simulink model "FinalTest_21_3_Duy"  (R2019b)
settings: Solver=VariableStepAuto  StartTime=0.0  StopTime=10.0  RelTol=1e-3
undefined symbols (not defined in the file): G, Rollingresistancecoefficient
libraries: simulink_extras x4, vehdynlibsteering x1, autolibshared x1
settings Model: Creator=Lenovo  LastModifiedBy=Lenovo
settings DebuggingCC: UnconnectedInputMsg=none  UnconnectedOutputMsg=none  UnconnectedLineMsg=none  SFMachineParentedDataDiag=error
settings ModelReferenceCC: EnableRefExpFcnMdlSchedulingChecks=off
settings RTWCC: Description=Generic Real-Time Target

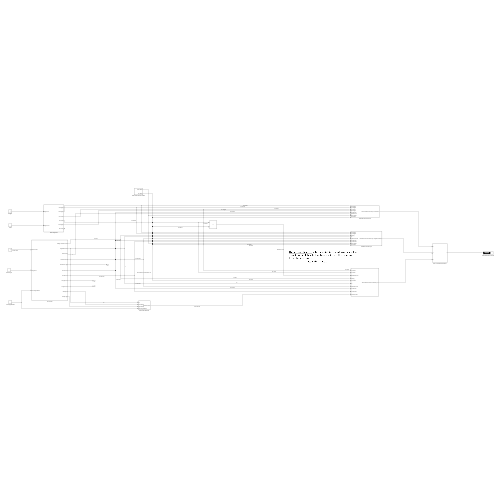
[thumbnail: Simulink's stored preview of the top-level diagram]
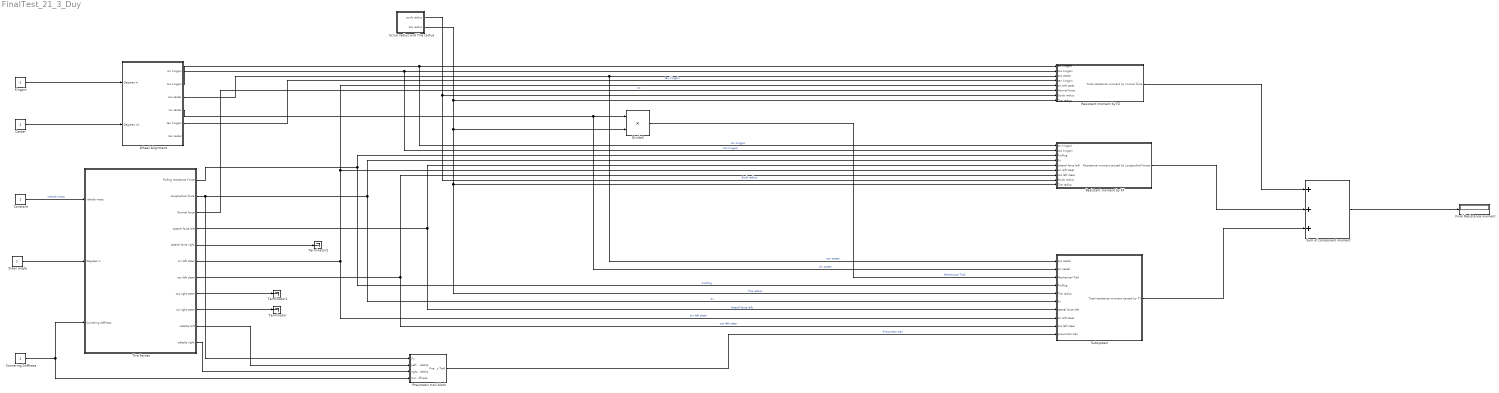
== system FinalTest_21_3_Duy ==
  Caster : Constant
  Constant : Constant
  Cornering Stiffness : Constant
  Divide2 : Product  Inputs=**
  Final Resistance moment : Display
  Kingpin : Constant
  Pneumatic trail block : Subsystem
  Resistant moment by FX : Subsystem
  Resistant moment by FZ : Subsystem
  Scrub radius and Tire radius : Subsystem
  Steer angle : Constant
  Subsystem : Subsystem
  Sum of component moment : Sum  Inputs=+++
  Terminator : Terminator
  Terminator1 : Terminator
  Terminator2 : Terminator
  Tire Forces : Subsystem
  Wheel Alignment : Subsystem
  wires:
  Constant/1 -> Tire Forces/1(vehicle mass)  "vehicle mass"
  Steer angle/1 -> Tire Forces/2(Degrees in)
  Tire Forces/3(Normal force) -> Resistant moment by FZ/6(Normal force)  "Fz"
  Tire Forces/5(Lateral force right) -> Terminator2/1
  Tire Forces/8(cos right steer) -> Terminator1/1
  Tire Forces/9(sin right steer) -> Terminator/1
  Kingpin/1 -> Wheel Alignment/1(Degrees in)
  Caster/1 -> Wheel Alignment/2(Degrees in1)
  Wheel Alignment/4(sin caster) -> Subsystem/2(sin caster), Divide2/1  "sin caster"
  Wheel Alignment/1(sin kingpin) -> Resistant moment by FX/1(sin kingpin), Resistant moment by FZ/1(sin kingpin)  "sin kingpin"
  Wheel Alignment/2(cos kingpin) -> Resistant moment by FX/2(cos kingpin), Resistant moment by FZ/2(cos kingpin)  "cos kingpin"
  Wheel Alignment/3(cos caster) -> Subsystem/1(cos caster), Resistant moment by FZ/3(cos caster)  "cos caster"
  Wheel Alignment/5(tan kingpin) -> Resistant moment by FZ/4(tan kingpin)  "tan kingpin"
  Tire Forces/6(sin left steer) -> Subsystem/8(sin left steer), Resistant moment by FZ/5(sin left steer), Resistant moment by FX/6(sin left steer)  "sin left steer"
  Tire Forces/1(Rolling resistance Force) -> Subsystem/4(Frolling), Resistant moment by FX/3(Frolling)  "Frolling"
  Tire Forces/2(Longitudinal force) -> Pneumatic trail block/1(Fx), Subsystem/6(Fx), Resistant moment by FX/4(Fx)  "Fx"
  Tire Forces/4(Lateral force left) -> Subsystem/7(lateral force left), Resistant moment by FX/5(Lateral force left)  "lateral force left"
  Tire Forces/7(cos left steer) -> Subsystem/9(cos left steer), Resistant moment by FX/7(cos left steer)  "cos left steer"
  Cornering Stiffness/1 -> Pneumatic trail block/4(Cornering Stiffness), Tire Forces/3(Cornering stiffness)
  Tire Forces/10(sidelsip left) -> Pneumatic trail block/2(Left sideslip)
  Tire Forces/11(sideslip right) -> Pneumatic trail block/3(right sideslip)
  Scrub radius and Tire radius/2(tire radius) -> Subsystem/5(Tire radius), Resistant moment by FX/9(Tire radius), Divide2/2, Resistant moment by FZ/8(Tire radius)  "Tire radius"
  Scrub radius and Tire radius/1(scrub radius) -> Resistant moment by FX/8(Scrub radius), Resistant moment by FZ/7(Scrub radius)  "Scub radius"
  Divide2/1 -> Subsystem/3(Mechanical Trail)  "Mechanical Trail"
  Pneumatic trail block/1(Pneumatic Trail) -> Subsystem/10(pneumatic trail)  "Pneumatic trail"
  Resistant moment by FZ/1(Toral resistance moment by normal force) -> Sum of component moment/1
  Subsystem/1(Total resistance moment caused by FY) -> Sum of component moment/3
  Resistant moment by FX/1(Resistance moment caused by Longitudinal forces) -> Sum of component moment/2
  Sum of component moment/1 -> Final Resistance moment/1

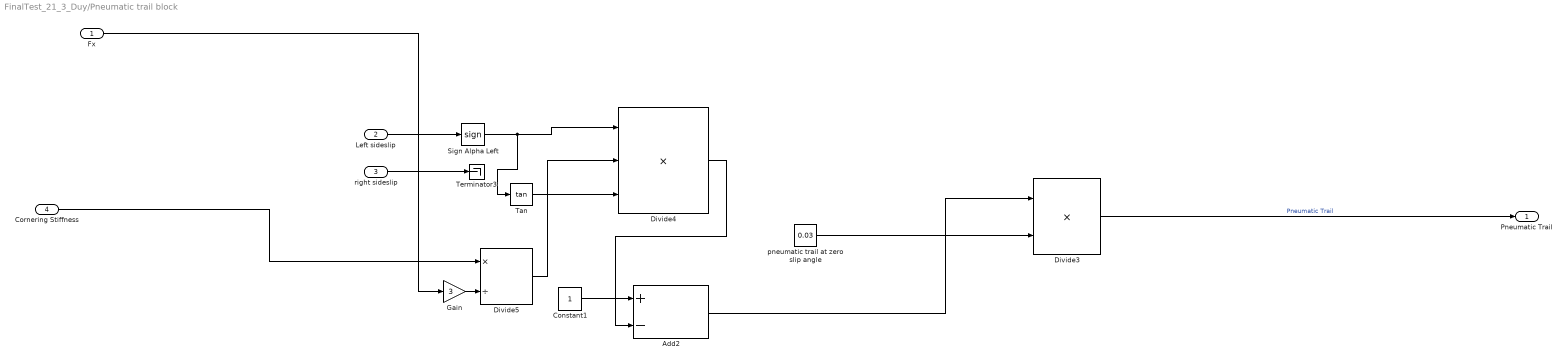
== system FinalTest_21_3_Duy/Pneumatic trail block ==
  Fx : Inport
  Left sideslip : Inport  Port=2
  right sideslip : Inport  Port=3
  Cornering Stiffness : Inport  Port=4
  Add2 : Sum  Inputs=+-
  Constant1 : Constant
  Divide3 : Product  Inputs=**
  Divide4 : Product  Inputs=***
  Divide5 : Product  Inputs=*/
  Gain : Gain  Gain=3
  Sign Alpha Left : Signum
  Tan : Trigonometry  Operator=tan
  Terminator3 : Terminator
  pneumatic trail at zero slip angle : Constant  Value=0.03
  Pneumatic Trail : Outport
  wires:
  Constant1/1 -> Add2/1
  Divide4/1 -> Add2/2
  Divide5/1 -> Divide4/2
  Tan/1 -> Divide4/3
  Sign Alpha Left/1 -> Tan/1, Divide4/1
  pneumatic trail at zero slip angle/1 -> Divide3/2
  Gain/1 -> Divide5/2
  Add2/1 -> Divide3/1
  Left sideslip/1 -> Sign Alpha Left/1
  Divide3/1 -> Pneumatic Trail/1  "Pneumatic Trail"
  right sideslip/1 -> Terminator3/1
  Fx/1 -> Gain/1
  Cornering Stiffness/1 -> Divide5/1

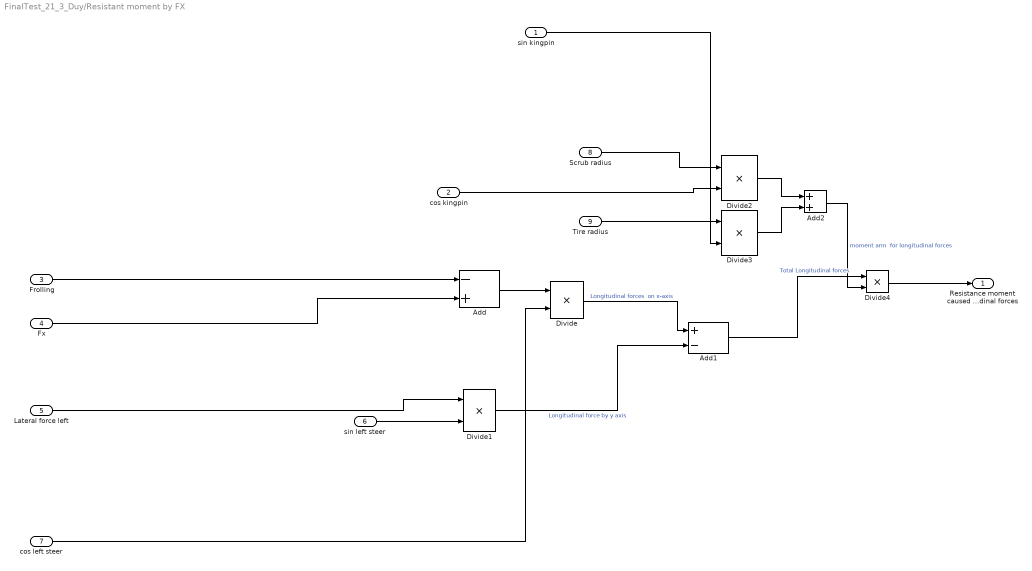
== system FinalTest_21_3_Duy/Resistant moment by FX ==
  sin kingpin : Inport
  cos kingpin : Inport  Port=2
  Frolling : Inport  Port=3
  Fx : Inport  Port=4
  Lateral force left : Inport  Port=5
  sin left steer : Inport  Port=6
  cos left steer : Inport  Port=7
  Scrub radius : Inport  Port=8
  Tire radius : Inport  Port=9
  Add : Sum  Inputs=-+
  Add1 : Sum  Inputs=+-
  Add2 : Sum
  Divide{,1..4} (5 alike) : Product  Inputs=**
  Resistance moment caused by Longitudinal forces : Outport
  wires:
  Scrub radius/1 -> Divide2/1
  Add1/1 -> Divide4/1  "Total Longitudinal forces"
  Divide/1 -> Add1/1  "Longitudinal forces  on x-axis"
  Divide1/1 -> Add1/2  "Longitudinal force by y axis"
  Lateral force left/1 -> Divide1/1
  Add/1 -> Divide/1
  Add2/1 -> Divide4/2  "moment arm  for longitudinal forces"
  Divide4/1 -> Resistance moment caused by Longitudinal forces/1
  Divide2/1 -> Add2/1
  Tire radius/1 -> Divide3/1
  Divide3/1 -> Add2/2
  cos kingpin/1 -> Divide2/2
  cos left steer/1 -> Divide/2
  sin left steer/1 -> Divide1/2
  Fx/1 -> Add/2
  Frolling/1 -> Add/1
  sin kingpin/1 -> Divide3/2

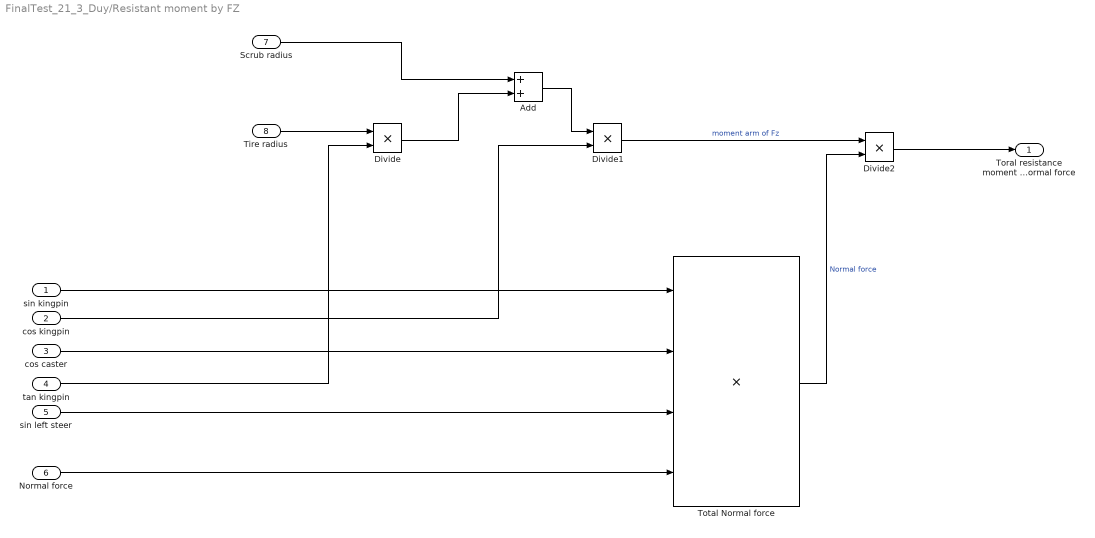
== system FinalTest_21_3_Duy/Resistant moment by FZ ==
  sin kingpin : Inport
  cos kingpin : Inport  Port=2
  cos caster : Inport  Port=3
  tan kingpin : Inport  Port=4
  sin left steer : Inport  Port=5
  Normal force : Inport  Port=6
  Scrub radius : Inport  Port=7
  Tire radius : Inport  Port=8
  Add : Sum
  Divide : Product  Inputs=**
  Divide1 : Product  Inputs=**
  Divide2 : Product  Inputs=**
  Total Normal force : Product  Inputs=****
  Toral resistance moment by normal force : Outport
  wires:
  Tire radius/1 -> Divide/1
  cos kingpin/1 -> Divide1/2
  sin kingpin/1 -> Total Normal force/1
  Scrub radius/1 -> Add/1
  Total Normal force/1 -> Divide2/2  "Normal force"
  Divide1/1 -> Divide2/1  "moment arm of Fz"
  Divide/1 -> Add/2
  Add/1 -> Divide1/1
  cos caster/1 -> Total Normal force/2
  sin left steer/1 -> Total Normal force/3
  tan kingpin/1 -> Divide/2
  Divide2/1 -> Toral resistance moment by normal force/1
  Normal force/1 -> Total Normal force/4

== system FinalTest_21_3_Duy/Scrub radius and Tire radius ==
  Scrub radius : Constant
  Tire radius : Constant
  scrub radius : Outport
  tire radius : Outport  Port=2
  wires:
  Tire radius/1 -> tire radius/1  "tire radius"
  Scrub radius/1 -> scrub radius/1  "scrub radius"

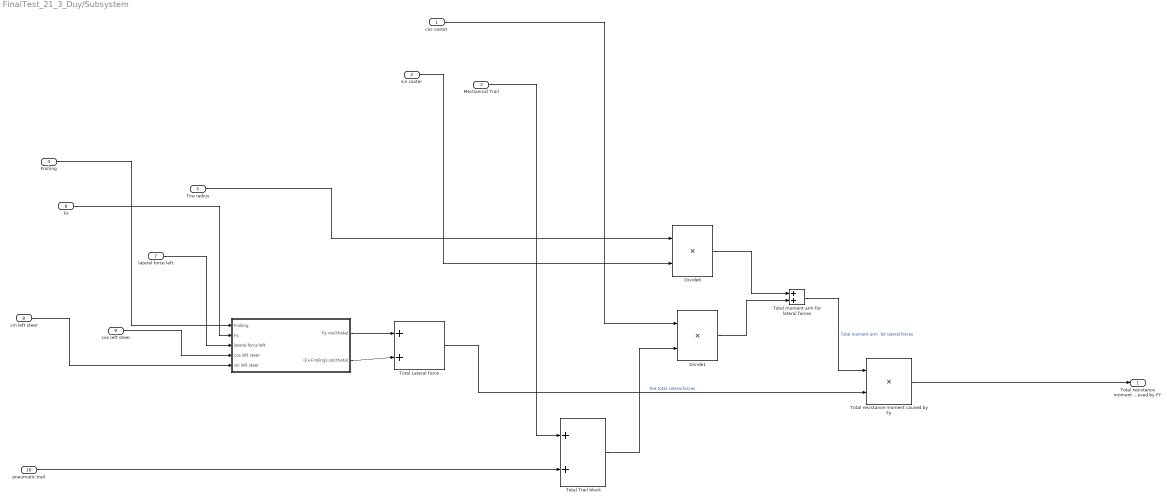
== system FinalTest_21_3_Duy/Subsystem ==
  cos caster : Inport
  sin caster : Inport  Port=2
  Mechanical Trail : Inport  Port=3
  Frolling : Inport  Port=4
  Tire radius : Inport  Port=5
  Fx : Inport  Port=6
  lateral force left : Inport  Port=7
  sin left steer : Inport  Port=8
  cos left steer : Inport  Port=9
  pneumatic trail : Inport  Port=10
  " " : Subsystem
  Divide1 : Product  Inputs=**
  Divide6 : Product  Inputs=**
  Total Lateral force : Sum
  Total Trail block : Sum
  Total moment arm for lateral forces : Sum
  Total resistance moment caused by Fy : Product  Inputs=**
  Total resistance moment caused by FY : Outport
  wires:
  cos caster/1 -> Divide1/1
  Divide6/1 -> Total moment arm for lateral forces/1
  Total moment arm for lateral forces/1 -> Total resistance moment caused by Fy/1  "Total moment arm  for lateral forces"
  Total Lateral force/1 -> Total resistance moment caused by Fy/2  "the total  lateral forces"
  Divide1/1 -> Total moment arm for lateral forces/2
  " "/1(Fy.cos(theta)) -> Total Lateral force/1
  Total Trail block/1 -> Divide1/2
  " "/2((Fx-Frolling).sin(theta)) -> Total Lateral force/2
  Total resistance moment caused by Fy/1 -> Total resistance moment caused by FY/1
  pneumatic trail/1 -> Total Trail block/2
  Tire radius/1 -> Divide6/1
  sin caster/1 -> Divide6/2
  cos left steer/1 -> " "/4(cos left steer)
  Frolling/1 -> " "/1(Frolling)
  lateral force left/1 -> " "/3(lateral force left)
  sin left steer/1 -> " "/5(sin left steer)
  Fx/1 -> " "/2(Fx)
  Mechanical Trail/1 -> Total Trail block/1

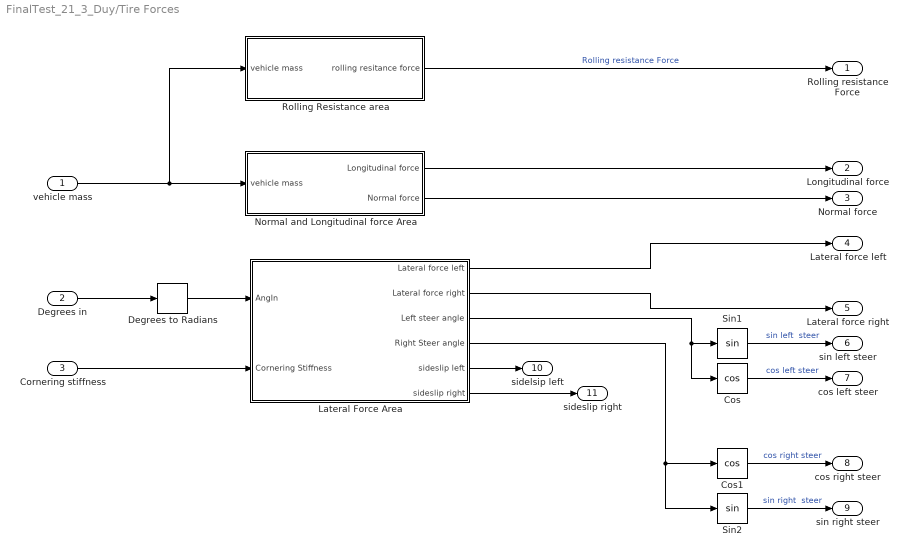
== system FinalTest_21_3_Duy/Tire Forces ==
  vehicle mass : Inport
  Degrees in : Inport  Port=2
  Cornering stiffness : Inport  Port=3
  Cos : Trigonometry  Operator=cos
  Cos1 : Trigonometry  Operator=cos
  Degrees to Radians : simulink_extras/Transformations/Degrees to Radians
  Lateral Force Area : Subsystem
  Normal and Longitudinal force Area : Subsystem
  Rolling Resistance area : Subsystem
  Sin1 : Trigonometry
  Sin2 : Trigonometry
  Rolling resistance Force : Outport
  Longitudinal force : Outport  Port=2
  Normal force : Outport  Port=3
  Lateral force left : Outport  Port=4
  Lateral force right : Outport  Port=5
  sin left steer : Outport  Port=6
  cos left steer : Outport  Port=7
  cos right steer : Outport  Port=8
  sin right steer : Outport  Port=9
  sidelsip left : Outport  Port=10
  sideslip right : Outport  Port=11
  wires:
  Degrees to Radians/1 -> Lateral Force Area/1(AngIn)
  Lateral Force Area/4(Right Steer angle) -> Sin2/1, Cos1/1
  vehicle mass/1 -> Rolling Resistance area/1(vehicle mass), Normal and Longitudinal force Area/1(vehicle mass)
  Sin2/1 -> sin right steer/1  "sin right  steer"
  Cos1/1 -> cos right steer/1  "cos right steer"
  Lateral Force Area/3(Left steer angle) -> Sin1/1, Cos/1
  Normal and Longitudinal force Area/1(Longitudinal force) -> Longitudinal force/1
  Normal and Longitudinal force Area/2(Normal force) -> Normal force/1
  Sin1/1 -> sin left steer/1  "sin left  steer"
  Rolling Resistance area/1(rolling resitance force) -> Rolling resistance Force/1  "Rolling resistance Force"
  Degrees in/1 -> Degrees to Radians/1
  Cos/1 -> cos left steer/1  "cos left steer"
  Lateral Force Area/2(Lateral force right) -> Lateral force right/1
  Lateral Force Area/1(Lateral force left) -> Lateral force left/1
  Lateral Force Area/5(sideslip left) -> sidelsip left/1
  Lateral Force Area/6("sideslip right ") -> sideslip right/1
  Cornering stiffness/1 -> Lateral Force Area/2(Cornering Stiffness)

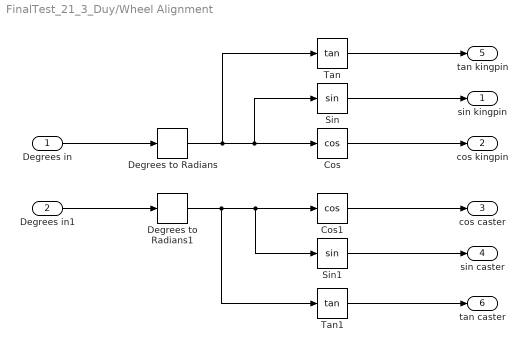
== system FinalTest_21_3_Duy/Wheel Alignment ==
  Degrees in : Inport
  Degrees in1 : Inport  Port=2
  Cos : Trigonometry  Operator=cos
  Cos1 : Trigonometry  Operator=cos
  Degrees to Radians : simulink_extras/Transformations/Degrees to Radians
  Degrees to Radians1 : simulink_extras/Transformations/Degrees to Radians
  Sin : Trigonometry
  Sin1 : Trigonometry
  Tan : Trigonometry  Operator=tan
  Tan1 : Trigonometry  Operator=tan
  sin kingpin : Outport
  cos kingpin : Outport  Port=2
  cos caster : Outport  Port=3
  sin caster : Outport  Port=4
  tan kingpin : Outport  Port=5
  tan caster : Outport  Port=6
  wires:
  Sin1/1 -> sin caster/1
  Degrees to Radians1/1 -> Tan1/1, Sin1/1, Cos1/1
  Sin/1 -> sin kingpin/1
  Degrees in1/1 -> Degrees to Radians1/1
  Cos1/1 -> cos caster/1
  Cos/1 -> cos kingpin/1
  Degrees to Radians/1 -> Tan/1, Sin/1, Cos/1
  Degrees in/1 -> Degrees to Radians/1
  Tan/1 -> tan kingpin/1
  Tan1/1 -> tan caster/1

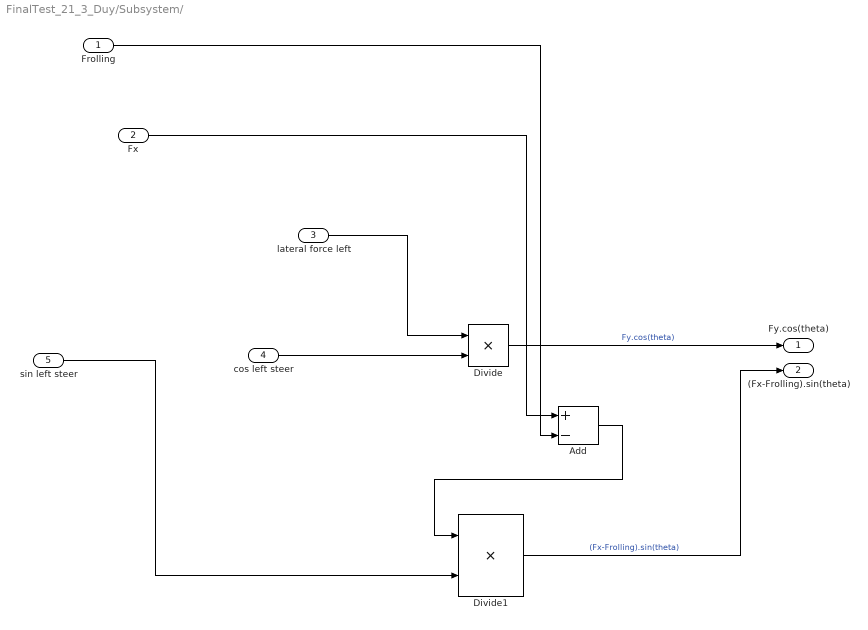
== system FinalTest_21_3_Duy/Subsystem/  ==
  Frolling : Inport
  Fx : Inport  Port=2
  lateral force left : Inport  Port=3
  cos left steer : Inport  Port=4
  sin left steer : Inport  Port=5
  Add : Sum  Inputs=+-
  Divide : Product  Inputs=**
  Divide1 : Product  Inputs=**
  Fy.cos(theta) : Outport
  (Fx-Frolling).sin(theta) : Outport  Port=2
  wires:
  Divide1/1 -> (Fx-Frolling).sin(theta)/1  "(Fx-Frolling).sin(theta)"
  Add/1 -> Divide1/1
  Frolling/1 -> Add/2
  lateral force left/1 -> Divide/1
  cos left steer/1 -> Divide/2
  sin left steer/1 -> Divide1/2
  Fx/1 -> Add/1
  Divide/1 -> Fy.cos(theta)/1  "Fy.cos(theta)"

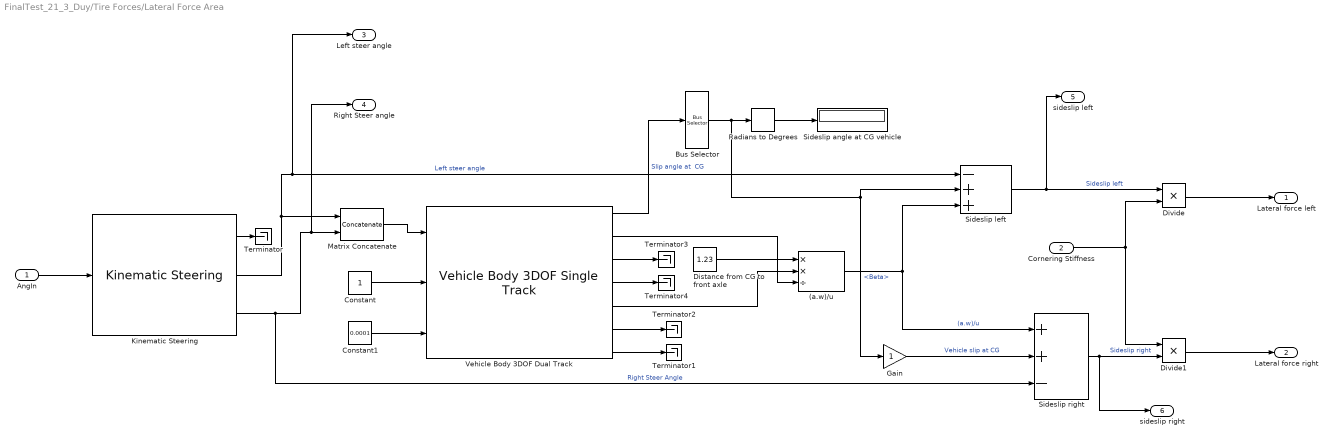
== system FinalTest_21_3_Duy/Tire Forces/Lateral Force Area ==
  AngIn : Inport
  Cornering Stiffness : Inport  Port=2
  (a.w)/u : Product  Inputs=**/
  Bus Selector : BusSelector  OutputSignals=BdyFrm.Cg.Ang.Beta
  Constant : Constant
  Constant1 : Constant  Value=0.0001
  Distance from CG to front axle : Constant  Value=1.23
  Divide : Product  Inputs=**
  Divide1 : Product  Inputs=**
  Gain : Gain
  Kinematic Steering : vehdynlibsteering/Kinematic Steering  StrgType=Rack and pinion  StrgRatioType=Constant  Loc=Front  NrmlFctr=0.01  TrckWdth=1.475  WhlBase=1.524  Db=0  StrgRng=6*pi  StrgAngBpts="[-6.2832   -5.0265   -3.7699   -2.5133   -1.2566         0    1.2566    2.5133    3.7699    5.0265    6.2832]"  StrgRatioTbl=|  StrgRatio=100  PctAckIn=off  PctAck=100  PctAckTbl=ones(1,11)*100  StrgArmLngth=0.3  RckCsLngth=0.65  TieRodLngth=0.13  D=0.12  PnnRadius=0.007  PnnRadiusTbl="[0.0055    0.0055    0.0056    0.0057    0.0058    0.0057    0.0057    0.0057    0.0056    0.0055    0.0055]"  RodLngth=0.1  ParaArmLngth=0.9  aMode=2
      | [13.5000   13.3750   13.2500   13.1250   13.0000   13.0000   13.0000   13.1250   13.2500   13.3750   13.5000
      | ]
  Matrix Concatenate : Concatenate  ConcatenateDimension=2
  Radians to Degrees : simulink_extras/Transformations/Radians to Degrees
  Sideslip angle at CG vehicle : Display
  Sideslip left : Sum  Inputs=-++
  Sideslip right : Sum  Inputs=++-
  Terminator{,1..4} (5 alike) : Terminator
  Vehicle Body 3DOF Dual Track : autolibshared/Vehicle Body 3DOF Single Track  trackMode=Dual  inputMode=External longitudinal velocity  frontSteerMode=on  rearSteerMode=off  windMode=off  muMode=off  extFMode=off  extMMode=off  htchFMode=off  htchMMode=off  extXo=off  extpsio=off  extxdoto=off  extro=off  extYo=off  extTamb=off  extydoto=on  aMode=2  NF=2  NR=2  m=2000  a=1.23  b=1.46  h=0.35  dh=1  hh=0.2  X_o=0  xdot_o=0  CalphaMode=off  sigmaMode=on  d=0  hl=0  w=[1.4,1.4]  Cy_f=52000  Cy_r=64000  sigma_f=.1  sigma_r=.1  alpha_f_brk=[-.1 .1]  Cy_f_data=[-9e3 9e3]  alpha_r_brk=[-.1 .1]  Cy_r_data=[-9e3 9e3]  Y_o=0  ydot_o=0  Izz=3600  psi_o=0  r_o=0  Af=2  Cd=.3  Cl=.1  Cpm=.1  beta_w=[0 0.01:0.01:0.3]  Cs=[0:0.03:0.9]  Cym=[0 1e-6:0.01:0.3]  Pabs=101325  Tair=273  g=9.81  mu=1  xdot_tol=.01  Fznom=5000  Fxtire_sat=7e4  Fytire_sat=7e4  longOff=0  latOff=0  vertOff=0  wrapAng=off
  Lateral force left : Outport
  Lateral force right : Outport  Port=2
  Left steer angle : Outport  Port=3
  Right Steer angle : Outport  Port=4
  sideslip left : Outport  Port=5
  "sideslip right " : Outport  Port=6
  wires:
  Radians to Degrees/1 -> Sideslip angle at CG vehicle/1
  Sideslip right/1 -> "sideslip right "/1, Divide1/2  "Sideslip right"
  Vehicle Body 3DOF Dual Track/4 -> Terminator4/1
  Vehicle Body 3DOF Dual Track/6 -> Terminator2/1
  Kinematic Steering/2 -> Left steer angle/1, Sideslip left/1, Matrix Concatenate/1  "Left steer angle"
  (a.w)/u/1 -> Sideslip right/1, Sideslip left/3  "(a.w)/u"
  Gain/1 -> Sideslip right/2  "Vehicle slip at CG"
  Distance from CG to front axle/1 -> (a.w)/u/1
  Matrix Concatenate/1 -> Vehicle Body 3DOF Dual Track/1
  Bus Selector/1 -> Gain/1, Sideslip left/2, Radians to Degrees/1  "<Beta>"
  Cornering Stiffness/1 -> Divide1/1, Divide/2
  Constant/1 -> Vehicle Body 3DOF Dual Track/2
  Constant1/1 -> Vehicle Body 3DOF Dual Track/3
  Kinematic Steering/1 -> Terminator/1
  Vehicle Body 3DOF Dual Track/2 -> (a.w)/u/3
  Vehicle Body 3DOF Dual Track/1 -> Bus Selector/1  "Slip angle at  CG"
  Vehicle Body 3DOF Dual Track/3 -> Terminator3/1
  Kinematic Steering/3 -> Sideslip right/3, Right Steer angle/1, Matrix Concatenate/2  "Right Steer Angle"
  Divide1/1 -> Lateral force right/1
  Sideslip left/1 -> sideslip left/1, Divide/1  "Sideslip left"
  AngIn/1 -> Kinematic Steering/1
  Vehicle Body 3DOF Dual Track/5 -> (a.w)/u/2
  Vehicle Body 3DOF Dual Track/7 -> Terminator1/1
  Divide/1 -> Lateral force left/1

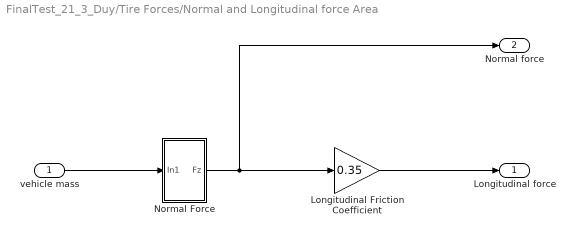
== system FinalTest_21_3_Duy/Tire Forces/Normal and Longitudinal force Area ==
  vehicle mass : Inport
  Longitudinal Friction Coefficient : Gain  Gain=0.35
  Normal Force : Subsystem
  Longitudinal force : Outport
  Normal force : Outport  Port=2
  wires:
  Normal Force/1(Fz) -> Normal force/1, Longitudinal Friction Coefficient/1
  Longitudinal Friction Coefficient/1 -> Longitudinal force/1
  vehicle mass/1 -> Normal Force/1(In1)

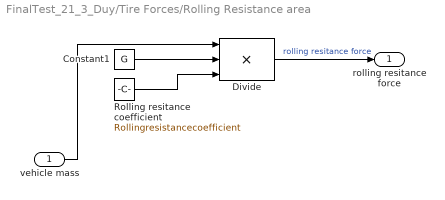
== system FinalTest_21_3_Duy/Tire Forces/Rolling Resistance area ==
  vehicle mass : Inport
  Constant1 : Constant  Value=G
  Divide : Product  Inputs=***
  Rolling resitance coefficient : Constant  Value=Rollingresistancecoefficient
  rolling resitance force : Outport
  wires:
  Rolling resitance coefficient/1 -> Divide/3
  Constant1/1 -> Divide/2
  Divide/1 -> rolling resitance force/1  "rolling resitance force"
  vehicle mass/1 -> Divide/1

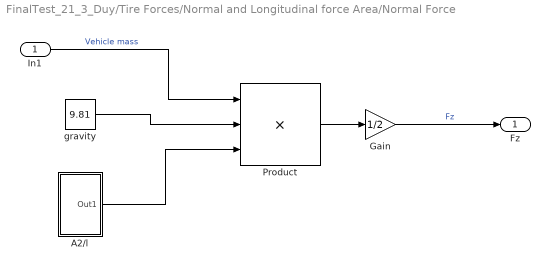
== system FinalTest_21_3_Duy/Tire Forces/Normal and Longitudinal force Area/Normal Force ==
  In1 : Inport
  A2/l : Subsystem
  Gain : Gain  Gain=1/2
  Product : Product  Inputs=3
  gravity : Constant  Value=9.81
  Fz : Outport
  wires:
  Gain/1 -> Fz/1  "Fz"
  Product/1 -> Gain/1
  gravity/1 -> Product/2
  A2/l/1(Out1) -> Product/3
  In1/1 -> Product/1  "Vehicle mass"

== system FinalTest_21_3_Duy/Tire Forces/Normal and Longitudinal force Area/Normal Force/A2//l ==
  Divide : Product  Inputs=*/
  Length from CG to rear axle : Constant  Value=4
  Wheelbase : Constant  Value=2
  Out1 : Outport
  wires:
  Wheelbase/1 -> Divide/2
  Length from CG to rear axle/1 -> Divide/1
  Divide/1 -> Out1/1
